simulink model "Q19"  (Simulink 9.1)
settings: Solver=VariableStepAuto  StartTime=0.0  StopTime=500  RelTol=1e-3
settings Model: Creator=GamePC  LastModifiedBy=GamePC
settings DataIOCC: SaveFormat=Dataset
settings OptimizationCC: LifeSpan=auto
settings DebuggingCC: UnderspecifiedInitializationDetection=Simplified  MergeDetectMultiDrivingBlocksExec=error  SFUnexpectedBacktrackingDiag=error  SFNoUnconditionalDefaultTransitionDiag=error  SFExecutionAtInitializationDiag=warning
settings HardwareCC: ProdBitPerPointer=64  ProdBitPerSizeT=64  ProdBitPerPtrDiffT=64  ProdLargestAtomicFloat=Float  ProdIntDivRoundTo=Zero  ProdEndianess=LittleEndian  ProdWordSize=64  ProdHWDeviceType=Intel->x86-64 (Windows64)
settings ModelReferenceCC: PropagateSignalLabelsOutOfModel=on
settings CodeAppCC: StateflowObjectComments=off
settings GRTTargetCC: TargetLangStandard=C99 (ISO)  CombineOutputUpdateFcns=on  GRTInterface=off
settings ConfigComp: CovMetricSettings=dwe  CovHtmlReporting=off  CovSaveCumulativeToWorkspaceVar=off  CovSaveSingleToWorkspaceVar=off  CovExternalEMLEnable=on

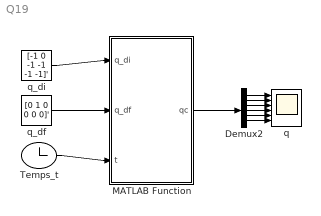
== system Q19 ==
  Demux2 : Demux  Outputs=6
  MATLAB Function : MATLAB Function  TreatAsAtomicUnit=on
  "Temps_t " : Clock
  q : Scope  NumInputPorts=6
  "q_df " : Constant  Value=[0 1 0 0 0 0]'  VectorParams1D=off
  q_di : Constant  Value=[-1 0 -1 -1 -1 -1]'  VectorParams1D=off
  wires:
  q_di/1 -> MATLAB Function/1(q_di)
  "q_df "/1 -> MATLAB Function/2(q_df)
  "Temps_t "/1 -> MATLAB Function/3(t)
  MATLAB Function/1(qc) -> Demux2/1
  Demux2/1 -> q/1
  Demux2/3 -> q/3
  Demux2/5 -> q/5
  Demux2/4 -> q/4
  Demux2/2 -> q/2
  Demux2/6 -> q/6

== matlab function MATLAB Function ==
  data: q_di input double; qc output double; q_df input double; t input double
function qc = GenTraj(q_di, q_df, t)
    
    tf = 500; % ms     
    D = (q_df - q_di);    
    r = 10 * (t/tf)^3 - 15 * (t/tf)^4 + 6 * (t/tf)^5;   
    qc = q_di + r*D;
end
